simulink model "Simulink0Ejemplo"  (R2021a)
settings: Solver=VariableStepAuto  StartTime=0.0  StopTime=10.0  RelTol=1e-3
undefined symbols (not defined in the file or in its folder): DiscIntNeverNeededParam
settings Model: Creator=agher  LastModifiedBy=agher

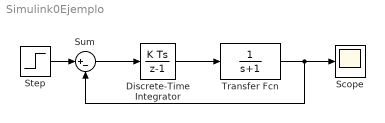
== system Simulink0Ejemplo ==
  Discrete-Time Integrator : DiscreteIntegrator  SampleTime=.01  ICPrevOutput=DiscIntNeverNeededParam  ICPrevScaledInput=DiscIntNeverNeededParam
  Scope : Scope
  Step : Step  SampleTime=0
  Sum : Sum  Inputs=|+-
  Transfer Fcn : TransferFcn  Denominator=[1 1]
  wires:
  Discrete-Time Integrator/1 -> Transfer Fcn/1
  Sum/1 -> Discrete-Time Integrator/1
  Transfer Fcn/1 -> Scope/1, Sum/2
  Step/1 -> Sum/1
